simulink model "OFDM_Tx_Rx_InterpDec"  (R2020a)
settings: Solver=FixedStepDiscrete  StartTime=0.0  StopTime=inf  RelTol=1e-3
InitFcn:
  | % Set parameters
  | fs = 200e3;
  | 
  | % Load all required variables
  | load('read_addr_data');
  | load('read_addr_cp');
  | load('read_addr_pream');
  | load('read_addr_rx');
  | load('pilot');
  | load('LTSfreq');
  | load('STSfreq');
  | load('LTSread');
  | load('STSread');
  | load('bpsk');
  | load('qpsk');
  | load('qam16');
values from neighbouring files (symbols this model uses):
  bpsk = [0 0 1 1 1 1 0 0 1 0 1 0 ... (48 elements, 48x1)]    [bpsk.mat]
  qam16 = [12 5 10 3 14 8 1 10 8 7 2 13 ... (48 elements, 48x1)]    [qam16.mat]
  qpsk = [1 2 1 2 2 2 3 1 1 3 1 0 ... (48 elements, 48x1)]    [qpsk.mat]
  STSfreq = [0 0 0 0 0 0 0 0 1 0 0 0 ... (64 elements, 1x64)]    [STSfreq.mat]
undefined symbols (not defined in the file or in its folder): data3, designMultirateFIR, LTSfreq, LTSread, pilot, read_addr_cp, read_addr_data, read_addr_pream, read_addr_rx, STSread
libraries: hdlsllib x58, simulink x42, dspmlti4 x8, dsphdlxfrm x2, dsphdlmathfun x2, dsphdlsigops x1
(part 3 of 5)

== system OFDM_Tx_Rx_InterpDec/OFDMRx/Synchronisation/ControlSigGen/dataValidGen ==
  enb : Inport
  enb1 : Inport  Port=2
  AND : Logic  IconShape=distinctive  AllPortsSameDT=off  OutDataTypeStr=boolean
  Compare To Constant : simulink/Logic and Bit Operations/Compare To Constant  relop=>  const=15  OutDataTypeStr=boolean
  Delay : Delay  DelayLength=1
  HDL Counter : hdlsllib/Sources/HDL Counter  CountType=Count limited  CountInit=0  CountStep=1  CountMax=79  CountFromType=Initial value  CountFrom=0  CountResetPort=on  CountLoadPort=off  CountEnbPort=on  CountDirPort=off  CountDataType=Unsigned  CountWordLen=7  CountFracLen=0  CountSampTime=1
  NOT : Logic  Operator=NOT  IconShape=distinctive  AllPortsSameDT=off  OutDataTypeStr=boolean
  NOT1 : Logic  Operator=NOT  IconShape=distinctive  AllPortsSameDT=off  OutDataTypeStr=boolean
  y : Outport
  wires:
  HDL Counter/1 -> Compare To Constant/1
  NOT/1 -> HDL Counter/1
  Compare To Constant/1 -> y/1
  NOT1/1 -> AND/1
  AND/1 -> NOT/1, HDL Counter/2
  Delay/1 -> AND/2
  enb1/1 -> Delay/1
  enb/1 -> NOT1/1

== system OFDM_Tx_Rx_InterpDec/OFDMRx/Synchronisation/FineTimingSynch/Abs1 ==
  DataIn : Inport
  Add : Sum  OutDataTypeStr=fixdt(1,16,14)
  Complex to Real-Imag : ComplexToRealImag
  Delay{,1..3} (4 alike) : Delay  DelayLength=1
  Product : Product
  Product1 : Product
  Out1 : Outport  VectorParamsAs1DForOutWhenUnconnected=off
  wires:
  Add/1 -> Out1/1
  Complex to Real-Imag/1 -> Delay/1
  DataIn/1 -> Complex to Real-Imag/1
  Product/1 -> Delay2/1
  Product1/1 -> Delay3/1
  Complex to Real-Imag/2 -> Delay1/1
  Delay/1 -> Product/1, Product/2
  Delay1/1 -> Product1/2, Product1/1
  Delay2/1 -> Add/1
  Delay3/1 -> Add/2

== system OFDM_Tx_Rx_InterpDec/OFDMRx/Synchronisation/FineTimingSynch/Abs2 ==
  dataOut : Inport
  Add : Sum
  Complex to Real-Imag : ComplexToRealImag
  Delay{,1..3} (4 alike) : Delay  DelayLength=1
  Gain : Gain  Gain=1/64  OutDataTypeStr=double
  Product : Product
  Product1 : Product
  Out1 : Outport  VectorParamsAs1DForOutWhenUnconnected=off
  wires:
  Delay3/1 -> Add/2
  Delay2/1 -> Add/1
  Delay1/1 -> Product1/1, Product1/2
  Delay/1 -> Product/2, Product/1
  Complex to Real-Imag/2 -> Delay1/1
  Product1/1 -> Delay3/1
  Product/1 -> Delay2/1
  Add/1 -> Gain/1
  dataOut/1 -> Complex to Real-Imag/1
  Complex to Real-Imag/1 -> Delay/1
  Gain/1 -> Out1/1

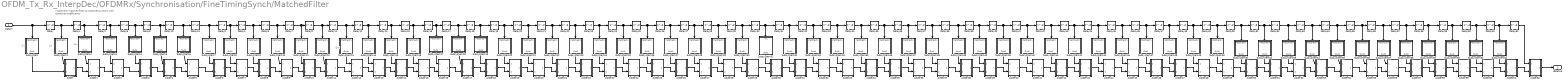
== system OFDM_Tx_Rx_InterpDec/OFDMRx/Synchronisation/FineTimingSynch/MatchedFilter ==
  note: -1+j
  note: 1+j
  note: 1-j
  note: -1-j
  note: Implement matched filter as pipleined systolic with
      | quantised coefficients
  dataIn : Inport
  Adder : Subsystem
  Adder1 : Subsystem
  Adder10 : Subsystem
  Adder11 : Subsystem
  Adder12 : Subsystem
  Adder13 : Subsystem
  Adder14 : Subsystem
  Adder15 : Subsystem
  Adder16 : Subsystem
  Adder17 : Subsystem
  Adder18 : Subsystem
  Adder19 : Subsystem
  Adder2 : Subsystem
  Adder20 : Subsystem
  Adder21 : Subsystem
  Adder22 : Subsystem
  Adder23 : Subsystem
  Adder24 : Subsystem
  Adder25 : Subsystem
  Adder26 : Subsystem
  Adder27 : Subsystem
  Adder28 : Subsystem
  Adder29 : Subsystem
  Adder3 : Subsystem
  Adder30 : Subsystem
  Adder31 : Subsystem
  Adder32 : Subsystem
  Adder33 : Subsystem
  Adder34 : Subsystem
  Adder35 : Subsystem
  Adder36 : Subsystem
  Adder37 : Subsystem
  Adder38 : Subsystem
  Adder39 : Subsystem
  Adder4 : Subsystem
  Adder40 : Subsystem
  Adder41 : Subsystem
  Adder42 : Subsystem
  Adder43 : Subsystem
  Adder44 : Subsystem
  Adder45 : Subsystem
  Adder46 : Subsystem
  Adder47 : Subsystem
  Adder48 : Subsystem
  Adder49 : Subsystem
  Adder5 : Subsystem
  Adder50 : Subsystem
  Adder51 : Subsystem
  Adder52 : Subsystem
  Adder53 : Subsystem
  Adder54 : Subsystem
  Adder55 : Subsystem
  Adder56 : Subsystem
  Adder57 : Subsystem
  Adder58 : Subsystem
  Adder59 : Subsystem
  Adder6 : Subsystem
  Adder60 : Subsystem
  Adder61 : Subsystem
  Adder62 : Subsystem
  Adder7 : Subsystem
  Adder8 : Subsystem
  Adder9 : Subsystem
  Delay{,1..62} (63 alike) : Delay
  Subsystem : Subsystem
  Subsystem1 : Subsystem
  Subsystem10 : Subsystem
  Subsystem11 : Subsystem
  Subsystem12 : Subsystem
  Subsystem13 : Subsystem
  Subsystem14 : Subsystem
  Subsystem15 : Subsystem
  Subsystem16 : Subsystem
  Subsystem17 : Subsystem
  Subsystem18 : Subsystem
  Subsystem19 : Subsystem
  Subsystem2 : Subsystem
  Subsystem20 : Subsystem
  Subsystem21 : Subsystem
  Subsystem22 : Subsystem
  Subsystem23 : Subsystem
  Subsystem24 : Subsystem
  Subsystem25 : Subsystem
  Subsystem26 : Subsystem
  Subsystem27 : Subsystem
  Subsystem28 : Subsystem
  Subsystem29 : Subsystem
  Subsystem3 : Subsystem
  Subsystem30 : Subsystem
  Subsystem31 : Subsystem
  Subsystem32 : Subsystem
  Subsystem33 : Subsystem
  Subsystem34 : Subsystem
  Subsystem35 : Subsystem
  Subsystem36 : Subsystem
  Subsystem37 : Subsystem
  Subsystem38 : Subsystem
  Subsystem39 : Subsystem
  Subsystem4 : Subsystem
  Subsystem40 : Subsystem
  Subsystem41 : Subsystem
  Subsystem42 : Subsystem
  Subsystem43 : Subsystem
  Subsystem44 : Subsystem
  Subsystem45 : Subsystem
  Subsystem46 : Subsystem
  Subsystem47 : Subsystem
  Subsystem48 : Subsystem
  Subsystem5 : Subsystem
  Subsystem50 : Subsystem
  Subsystem51 : Subsystem
  Subsystem52 : Subsystem
  Subsystem53 : Subsystem
  Subsystem54 : Subsystem
  Subsystem55 : Subsystem
  Subsystem56 : Subsystem
  Subsystem57 : Subsystem
  Subsystem58 : Subsystem
  Subsystem59 : Subsystem
  Subsystem6 : Subsystem
  Subsystem60 : Subsystem
  Subsystem61 : Subsystem
  Subsystem62 : Subsystem
  Subsystem63 : Subsystem
  Subsystem7 : Subsystem
  Subsystem8 : Subsystem
  Subsystem9 : Subsystem
  dataOut : Outport  VectorParamsAs1DForOutWhenUnconnected=off
  wires:
  Adder62/1(Out1) -> dataOut/1
  Adder61/1(Out1) -> Adder62/2(In2)
  Delay61/1 -> Subsystem62/1(MatchedIn), Delay62/1
  Adder60/1(Out1) -> Adder61/2(In2)
  Delay60/1 -> Subsystem61/1(MatchedIn), Delay61/1
  Adder59/1(Out1) -> Adder60/2(In2)
  Delay59/1 -> Delay60/1, Subsystem60/1(MatchedIn)
  Adder58/1(Out1) -> Adder59/2(In2)
  Delay58/1 -> Subsystem59/1(MatchedIn), Delay59/1
  Adder57/1(Out1) -> Adder58/2(In2)
  Delay57/1 -> Delay58/1, Subsystem58/1(MatchedIn)
  Adder56/1(Out1) -> Adder57/2(In2)
  Delay56/1 -> Subsystem57/1(MatchedIn), Delay57/1
  Adder55/1(Out1) -> Adder56/2(In2)
  Delay55/1 -> Subsystem56/1(MatchedIn), Delay56/1
  Adder54/1(Out1) -> Adder55/2(In2)
  Delay54/1 -> Subsystem55/1(MatchedIn), Delay55/1
  Adder53/1(Out1) -> Adder54/2(In2)
  Delay53/1 -> Subsystem54/1(MatchedIn), Delay54/1
  Adder52/1(Out1) -> Adder53/2(In2)
  Delay52/1 -> Subsystem53/1(MatchedIn), Delay53/1
  Adder51/1(Out1) -> Adder52/2(In2)
  Delay51/1 -> Delay52/1, Subsystem52/1(MatchedIn)
  Adder50/1(Out1) -> Adder51/2(In2)
  Delay50/1 -> Delay51/1, Subsystem51/1(MatchedIn)
  Adder49/1(Out1) -> Adder50/2(In2)
  Delay49/1 -> Delay50/1, Subsystem50/1(MatchedIn)
  Adder48/1(Out1) -> Adder49/2(In2)
  Delay48/1 -> Subsystem45/1(MatchedIn), Delay49/1
  Adder47/1(Out1) -> Adder48/2(In2)
  Delay47/1 -> Subsystem48/1(MatchedIn), Delay48/1
  Adder46/1(Out1) -> Adder47/2(In2)
  Delay46/1 -> Subsystem47/1(MatchedIn), Delay47/1
  Adder45/1(Out1) -> Adder46/2(In2)
  Delay45/1 -> Subsystem46/1(MatchedIn), Delay46/1
  Adder44/1(Out1) -> Adder45/2(In2)
  Delay44/1 -> Subsystem44/1(MatchedIn), Delay45/1
  Adder43/1(Out1) -> Adder44/2(In2)
  Delay43/1 -> Subsystem41/1(MatchedIn), Delay44/1
  Adder42/1(Out1) -> Adder43/2(In2)
  Delay42/1 -> Subsystem43/1(MatchedIn), Delay43/1
  Adder41/1(Out1) -> Adder42/2(In2)
  Delay41/1 -> Subsystem42/1(MatchedIn), Delay42/1
  Adder40/1(Out1) -> Adder41/2(In2)
  Delay40/1 -> Subsystem35/1(MatchedIn), Delay41/1
  Adder39/1(Out1) -> Adder40/2(In2)
  Delay39/1 -> Delay40/1, Subsystem40/1(MatchedIn)
  Adder38/1(Out1) -> Adder39/2(In2)
  Delay38/1 -> Subsystem39/1(MatchedIn), Delay39/1
  Adder37/1(Out1) -> Adder38/2(In2)
  Delay37/1 -> Delay38/1, Subsystem38/1(MatchedIn)
  Adder36/1(Out1) -> Adder37/2(In2)
  Delay36/1 -> Subsystem37/1(MatchedIn), Delay37/1
  Adder35/1(Out1) -> Adder36/2(In2)
  Delay35/1 -> Subsystem36/1(MatchedIn), Delay36/1
  Adder34/1(Out1) -> Adder35/2(In2)
  Delay34/1 -> Subsystem63/1(MatchedIn), Delay35/1
  Adder33/1(Out1) -> Adder34/2(In2)
  Delay33/1 -> Subsystem34/1(MatchedIn), Delay34/1
  Adder32/1(Out1) -> Adder33/2(In2)
  Delay32/1 -> Delay33/1, Subsystem33/1(MatchedIn)
  Adder31/1(Out1) -> Adder32/2(In2)
  Delay31/1 -> Subsystem32/1(MatchedIn), Delay32/1
  Adder30/1(Out1) -> Adder31/2(In2)
  Delay30/1 -> Subsystem31/1(In1), Delay31/1
  Adder29/1(Out1) -> Adder30/2(In2)
  Delay29/1 -> Delay30/1, Subsystem30/1(MatchedIn)
  Adder28/1(Out1) -> Adder29/2(In2)
  Delay28/1 -> Subsystem29/1(MatchedIn), Delay29/1
  Adder27/1(Out1) -> Adder28/2(In2)
  Delay27/1 -> Subsystem28/1(MatchedIn), Delay28/1
  Adder26/1(Out1) -> Adder27/2(In2)
  Delay26/1 -> Subsystem27/1(MatchedIn), Delay27/1
  Adder25/1(Out1) -> Adder26/2(In2)
  Delay25/1 -> Delay26/1, Subsystem26/1(MatchedIn)
  Adder24/1(Out1) -> Adder25/2(In2)
  Delay24/1 -> Subsystem25/1(MatchedIn), Delay25/1
  Adder23/1(Out1) -> Adder24/2(In2)
  Adder22/1(Out1) -> Adder23/2(In2)
  Delay21/1 -> Subsystem22/1(MatchedIn), Delay22/1
  Delay22/1 -> Subsystem23/1(MatchedIn), Delay23/1
  Adder21/1(Out1) -> Adder22/2(In2)
  Adder20/1(Out1) -> Adder21/2(In2)
  Delay20/1 -> Subsystem21/1(MatchedIn), Delay21/1
  Adder19/1(Out1) -> Adder20/2(In2)
  Delay19/1 -> Subsystem20/1(MatchedIn), Delay20/1
  Adder18/1(Out1) -> Adder19/2(In2)
  Adder17/1(Out1) -> Adder18/2(In2)
  Delay18/1 -> Subsystem19/1(MatchedIn), Delay19/1
  Delay17/1 -> Subsystem18/1(MatchedIn), Delay18/1
  Adder16/1(Out1) -> Adder17/2(In2)
  Adder15/1(Out1) -> Adder16/2(In2)
  Delay16/1 -> Subsystem17/1(MatchedIn), Delay17/1
  Delay15/1 -> Subsystem16/1(MatchedIn), Delay16/1
  Adder14/1(Out1) -> Adder15/2(In2)
  Adder13/1(Out1) -> Adder14/2(In2)
  Delay14/1 -> Subsystem15/1(MatchedIn), Delay15/1
  Adder12/1(Out1) -> Adder13/2(In2)
  Delay12/1 -> Subsystem14/1(MatchedIn), Delay14/1
  Adder11/1(Out1) -> Adder12/2(In2)
  Delay11/1 -> Subsystem13/1(MatchedIn), Delay12/1
  Adder10/1(Out1) -> Adder11/2(In2)
  Delay9/1 -> Subsystem12/1(MatchedIn), Delay11/1
  Adder9/1(Out1) -> Adder10/2(In2)
  Delay7/1 -> Subsystem11/1(MatchedIn), Delay9/1
  Delay5/1 -> Subsystem10/1(MatchedIn), Delay7/1
  Adder8/1(Out1) -> Adder9/2(In2)
  Adder7/1(Out1) -> Adder8/2(In2)
  Delay4/1 -> Subsystem9/1(MatchedIn), Delay5/1
  Adder6/1(Out1) -> Adder7/2(In2)
  Delay3/1 -> Subsystem8/1(MatchedIn), Delay4/1
  Adder5/1(Out1) -> Adder6/2(In2)
  Adder4/1(Out1) -> Adder5/2(In2)
  Adder3/1(Out1) -> Adder4/2(In2)
  Adder2/1(Out1) -> Adder3/2(In2)
  Adder1/1(Out1) -> Adder2/2(In2)
  Adder/1(Out1) -> Adder1/2(In2)
  Delay13/1 -> Subsystem7/1(MatchedIn), Delay3/1
  Delay10/1 -> Subsystem6/1(MatchedIn), Delay13/1
  Delay8/1 -> Subsystem5/1(MatchedIn), Delay10/1
  Delay6/1 -> Subsystem4/1(MatchedIn), Delay8/1
  Delay2/1 -> Subsystem3/1(MatchedIn), Delay6/1
  Delay1/1 -> Subsystem2/1(MatchedIn), Delay2/1
  Delay/1 -> Subsystem1/1(MatchedIn), Delay1/1
  dataIn/1 -> Delay/1, Subsystem/1(MatchedIn)
  Subsystem/1(Out1) -> Adder/2(In2)
  Subsystem1/1(Out1) -> Adder/1(In1)
  Subsystem3/1(Out1) -> Adder2/1(In1)
  Subsystem4/1(Out1) -> Adder3/1(In1)
  Subsystem5/1(Out1) -> Adder4/1(In1)
  Subsystem6/1(Out1) -> Adder5/1(In1)
  Subsystem7/1(Out1) -> Adder6/1(In1)
  Subsystem8/1(Out1) -> Adder7/1(In1)
  Subsystem9/1(Out1) -> Adder8/1(In1)
  Subsystem10/1(Out1) -> Adder9/1(In1)
  Subsystem11/1(Out1) -> Adder10/1(In1)
  Subsystem12/1(Out1) -> Adder11/1(In1)
  Subsystem13/1(Out1) -> Adder12/1(In1)
  Subsystem14/1(Out1) -> Adder13/1(In1)
  Subsystem15/1(Out1) -> Adder14/1(In1)
  Subsystem16/1(Out1) -> Adder15/1(In1)
  Subsystem17/1(Out1) -> Adder16/1(In1)
  Subsystem18/1(Out1) -> Adder17/1(In1)
  Subsystem19/1(Out1) -> Adder18/1(In1)
  Subsystem20/1(Out1) -> Adder19/1(In1)
  Subsystem21/1(Out1) -> Adder20/1(In1)
  Subsystem22/1(Out1) -> Adder21/1(In1)
  Subsystem23/1(Out1) -> Adder22/1(In1)
  Delay23/1 -> Subsystem24/1(MatchedIn), Delay24/1
  Subsystem24/1(Out1) -> Adder23/1(In1)
  Subsystem25/1(Out1) -> Adder24/1(In1)
  Subsystem26/1(Out1) -> Adder25/1(In1)
  Subsystem27/1(Out1) -> Adder26/1(In1)
  Subsystem28/1(Out1) -> Adder27/1(In1)
  Subsystem29/1(Out1) -> Adder28/1(In1)
  Subsystem30/1(Out1) -> Adder29/1(In1)
  Subsystem31/1(Out1) -> Adder30/1(In1)
  Subsystem32/1(Out1) -> Adder31/1(In1)
  Subsystem33/1(Out1) -> Adder32/1(In1)
  Subsystem34/1(Out1) -> Adder33/1(In1)
  Subsystem63/1(Out1) -> Adder34/1(In1)
  Subsystem36/1(Out1) -> Adder35/1(In1)
  Subsystem37/1(Out1) -> Adder36/1(In1)
  Subsystem38/1(Out1) -> Adder37/1(In1)
  Subsystem39/1(Out1) -> Adder38/1(In1)
  Subsystem40/1(Out1) -> Adder39/1(In1)
  Subsystem35/1(Out1) -> Adder40/1(In1)
  Subsystem42/1(Out1) -> Adder41/1(In1)
  Subsystem43/1(Out1) -> Adder42/1(In1)
  Subsystem41/1(Out1) -> Adder43/1(In1)
  Subsystem44/1(Out1) -> Adder44/1(In1)
  Subsystem46/1(Out1) -> Adder45/1(In1)
  Subsystem47/1(Out1) -> Adder46/1(In1)
  Subsystem48/1(Out1) -> Adder47/1(In1)
  Subsystem45/1(Out1) -> Adder48/1(In1)
  Subsystem50/1(Out1) -> Adder49/1(In1)
  Subsystem51/1(Out1) -> Adder50/1(In1)
  Subsystem52/1(Out1) -> Adder51/1(In1)
  Subsystem53/1(Out1) -> Adder52/1(In1)
  Subsystem54/1(Out1) -> Adder53/1(In1)
  Subsystem55/1(Out1) -> Adder54/1(In1)
  Subsystem56/1(Out1) -> Adder55/1(In1)
  Subsystem57/1(Out1) -> Adder56/1(In1)
  Subsystem58/1(Out1) -> Adder57/1(In1)
  Subsystem59/1(Out1) -> Adder58/1(In1)
  Subsystem60/1(Out1) -> Adder59/1(In1)
  Subsystem61/1(Out1) -> Adder60/1(In1)
  Subsystem62/1(Out1) -> Adder61/1(In1)
  Delay62/1 -> Adder62/1(In1)
  Subsystem2/1(Out1) -> Adder1/1(In1)

== system OFDM_Tx_Rx_InterpDec/OFDMRx/Synchronisation/FineTimingSynch/MovingAvg ==
  DataIn : Inport
  Add : Sum  Inputs=-+  AccumDataTypeStr=fixdt(1,24,14)
  Add1 : Sum  AccumDataTypeStr=fixdt(1,24,14)
  Delay1 : Delay  DelayLength=64
  Delay2 : Delay  DelayLength=1
  Delay3 : Delay  DelayLength=1
  Delay4 : Delay  DelayLength=1
  Out1 : Outport  VectorParamsAs1DForOutWhenUnconnected=off
  wires:
  Delay3/1 -> Add/2, Delay1/1
  Add/1 -> Add1/2
  Delay1/1 -> Add/1
  DataIn/1 -> Delay3/1
  Add1/1 -> Delay2/1
  Delay2/1 -> Delay4/1, Add1/1
  Delay4/1 -> Out1/1

== system OFDM_Tx_Rx_InterpDec/OFDMRx/Synchronisation/FineTimingSynch/threshCompare ==
  In1 : Inport
  In2 : Inport  Port=2
  Constant1 : Constant  OutDataTypeStr=boolean  SampleTime=1/fs
  Constant2 : Constant  Value=0  OutDataTypeStr=boolean  SampleTime=1/fs
  Relational Operator : RelationalOperator  Operator=>  OutDataTypeStr=boolean  RndMeth=Simplest
  Unit Delay Enabled Resettable Synchronous : hdlsllib/Discrete/Unit Delay Enabled Resettable Synchronous  InitialCondition=0.0  SampleTime=-1
      settings: SourceProductBaseCode=SL
  Out1 : Outport
  wires:
  Constant1/1 -> Unit Delay Enabled Resettable Synchronous/1
  In1/1 -> Relational Operator/1
  Relational Operator/1 -> Unit Delay Enabled Resettable Synchronous/2
  Unit Delay Enabled Resettable Synchronous/1 -> Out1/1
  Constant2/1 -> Unit Delay Enabled Resettable Synchronous/3
  In2/1 -> Relational Operator/2

== system OFDM_Tx_Rx_InterpDec/OFDMRx/Synchronisation/FrameDetect/RsingEdge ==
  In1 : Inport
  Constant : Constant  OutDataTypeStr=boolean  SampleTime=1/fs
  Constant1 : Constant  Value=0  OutDataTypeStr=boolean  SampleTime=1/fs
  Delay : Delay  DelayLength=1
  Relational Operator : RelationalOperator  Operator=>  OutDataTypeStr=boolean  RndMeth=Nearest
  Unit Delay Enabled Resettable Synchronous : hdlsllib/Discrete/Unit Delay Enabled Resettable Synchronous  InitialCondition=0.0  SampleTime=-1
      settings: SourceProductBaseCode=SL
  Out1 : Outport  VectorParamsAs1DForOutWhenUnconnected=off
  wires:
  Relational Operator/1 -> Unit Delay Enabled Resettable Synchronous/2
  Delay/1 -> Relational Operator/2
  In1/1 -> Delay/1, Relational Operator/1
  Unit Delay Enabled Resettable Synchronous/1 -> Out1/1
  Constant/1 -> Unit Delay Enabled Resettable Synchronous/1
  Constant1/1 -> Unit Delay Enabled Resettable Synchronous/3

== system OFDM_Tx_Rx_InterpDec/OFDMRx/Synchronisation/SchmidlCoxMetric /Abs2 ==
  Abs2In : Inport
  Add : Sum  OutDataTypeStr=fixdt(0,25,23)
  Complex to Real-Imag : ComplexToRealImag
  Delay{1..4} (4 alike) : Delay  DelayLength=1
  Delay5 : Delay
  Product : Product  OutDataTypeStr=fixdt(0,25,23)
  Product1 : Product  OutDataTypeStr=fixdt(0,25,23)
  Abs2Out : Outport  VectorParamsAs1DForOutWhenUnconnected=off
  wires:
  Delay5/1 -> Abs2Out/1
  Delay4/1 -> Add/2
  Delay3/1 -> Add/1
  Delay2/1 -> Product1/1, Product1/2
  Delay1/1 -> Product/2, Product/1
  Add/1 -> Delay5/1
  Product1/1 -> Delay4/1
  Product/1 -> Delay3/1
  Complex to Real-Imag/2 -> Delay2/1
  Complex to Real-Imag/1 -> Delay1/1
  Abs2In/1 -> Complex to Real-Imag/1

== system OFDM_Tx_Rx_InterpDec/OFDMRx/Synchronisation/SchmidlCoxMetric /AutoCorr ==
  AcorrIn : Inport
  Delay : Delay  DelayLength=16
  Delay{1..5} (5 alike) : Delay  DelayLength=1
  Math Function : Math  Operator=conj  SignedPower=on  RndMeth=Zero  SaturateOnIntegerOverflow=on
  Product : Product  OutDataTypeStr=fixdt(1,25,23)
  AcorrOut : Outport  VectorParamsAs1DForOutWhenUnconnected=off
  wires:
  Delay5/1 -> Delay2/1
  Delay4/1 -> Product/2
  Delay3/1 -> Product/1
  Delay2/1 -> AcorrOut/1
  Delay1/1 -> Delay3/1, Delay/1
  Delay/1 -> Math Function/1
  Product/1 -> Delay5/1
  Math Function/1 -> Delay4/1
  AcorrIn/1 -> Delay1/1

== system OFDM_Tx_Rx_InterpDec/OFDMRx/Synchronisation/SchmidlCoxMetric /CIC_ma ==
  note: The averaging window is set to 64 samples i.e.
      | 4x repetitions of the L-STF. Using a larger averaging
      | window improves the coarse CFO estimate. This
      | approach leaves 6x L-STF repetitions for AGC convergence.
  In1 : Inport
  Add : Sum  Inputs=-+  AccumDataTypeStr=fixdt(1,33,23)
  Add1 : Sum  AccumDataTypeStr=fixdt(1,33,23)
  Data Type Conversion : DataTypeConversion  OutDataTypeStr=fixdt(1,18,16)
  Delay1 : Delay  DelayLength=48
  Delay2 : Delay  DelayLength=1
  Delay3 : Delay  DelayLength=1
  Delay4 : Delay  DelayLength=1
  Out1 : Outport  VectorParamsAs1DForOutWhenUnconnected=off
  wires:
  Data Type Conversion/1 -> Out1/1
  Delay4/1 -> Data Type Conversion/1
  Delay3/1 -> Delay1/1, Add/2
  Delay2/1 -> Add1/1, Delay4/1
  Add1/1 -> Delay2/1
  In1/1 -> Delay3/1
  Delay1/1 -> Add/1
  Add/1 -> Add1/2

== system OFDM_Tx_Rx_InterpDec/OFDMRx/Synchronisation/SchmidlCoxMetric /CIC_ma1 ==
  In1 : Inport
  Add : Sum  Inputs=-+  AccumDataTypeStr=fixdt(1,33,23)
  Add1 : Sum  AccumDataTypeStr=fixdt(1,33,23)
  Data Type Conversion : DataTypeConversion  OutDataTypeStr=fixdt(1,18,15)
  Delay1 : Delay  DelayLength=48
  Delay2 : Delay  DelayLength=1
  Delay3 : Delay  DelayLength=1
  Delay4 : Delay  DelayLength=1
  Out1 : Outport  VectorParamsAs1DForOutWhenUnconnected=off
  wires:
  Data Type Conversion/1 -> Out1/1
  Delay4/1 -> Data Type Conversion/1
  Delay3/1 -> Add/2, Delay1/1
  Add/1 -> Add1/2
  Delay1/1 -> Add/1
  In1/1 -> Delay3/1
  Add1/1 -> Delay2/1
  Delay2/1 -> Delay4/1, Add1/1

== system OFDM_Tx_Rx_InterpDec/OFDMRx/Synchronisation/SchmidlCoxMetric /MagPhase ==
  dataIn : Inport
  Complex to Magnitude-Angle HDL Optimized : dsphdlmathfun/Complex to Magnitude-Angle HDL Optimized  NumIterationsSource=Property  NumIterations=10  OutputFormat=Magnitude and angle  AngleFormat=Normalized  ScaleOutput=on  SimulateUsing=Code generation
      settings: SourceProductBaseCode=DS
  Constant : Constant  OutDataTypeStr=boolean  SampleTime=1/fs
  Data Type Conversion : DataTypeConversion  OutDataTypeStr=fixdt(1,18,16)
  Data Type Conversion1 : DataTypeConversion  OutDataTypeStr=fixdt(1,25,22)
  Terminator1 : Terminator
  Phase : Outport  VectorParamsAs1DForOutWhenUnconnected=off
  Mag : Outport  Port=2  VectorParamsAs1DForOutWhenUnconnected=off
  wires:
  Data Type Conversion1/1 -> Phase/1
  Data Type Conversion/1 -> Mag/1
  Complex to Magnitude-Angle HDL Optimized/2 -> Data Type Conversion1/1
  Complex to Magnitude-Angle HDL Optimized/3 -> Terminator1/1
  Complex to Magnitude-Angle HDL Optimized/1 -> Data Type Conversion/1
  dataIn/1 -> Complex to Magnitude-Angle HDL Optimized/1
  Constant/1 -> Complex to Magnitude-Angle HDL Optimized/2

== system OFDM_Tx_Rx_InterpDec/OFDMRx/Synchronisation/SchmidlCoxMetric /Sq ==
  In1 : Inport
  Delay : Delay  DelayLength=1
  Delay1 : Delay  DelayLength=1
  Product : Product
  Out1 : Outport  VectorParamsAs1DForOutWhenUnconnected=off
  wires:
  Delay1/1 -> Out1/1
  Delay/1 -> Product/2, Product/1
  Product/1 -> Delay1/1
  In1/1 -> Delay/1

== system OFDM_Tx_Rx_InterpDec/OFDMRx/Synchronisation/SchmidlCoxMetric /Sq1 ==
  In1 : Inport
  Delay : Delay  DelayLength=1
  Delay1 : Delay  DelayLength=1
  Product : Product
  Out1 : Outport  VectorParamsAs1DForOutWhenUnconnected=off
  wires:
  In1/1 -> Delay/1
  Product/1 -> Delay1/1
  Delay/1 -> Product/1, Product/2
  Delay1/1 -> Out1/1

== system OFDM_Tx_Rx_InterpDec/OFDMRx/Synchronisation/SchmidlCoxMetric /ThreshMult ==
  In1 : Inport
  ThreshMult : Gain  Gain=0.5  OutDataTypeStr=fixdt(1,33,23)
  Out1 : Outport  VectorParamsAs1DForOutWhenUnconnected=off
  wires:
  In1/1 -> ThreshMult/1
  ThreshMult/1 -> Out1/1

== system OFDM_Tx_Rx_InterpDec/OFDMTx/CPAdd/DataExtend/READ_CTRL2 ==
  In1 : Inport
  In2 : Inport  Port=2
  Constant : Constant  Value=0  OutDataTypeStr=fixdt(0,8,0)  SampleTime=1/fs
  Switch : Switch  Criteria=u2 ~= 0
  Out1 : Outport  VectorParamsAs1DForOutWhenUnconnected=off
  wires:
  Constant/1 -> Switch/3
  In2/1 -> Switch/2
  In1/1 -> Switch/1
  Switch/1 -> Out1/1

== system OFDM_Tx_Rx_InterpDec/OFDMTx/CPAdd/LTFExtend/LTFValidGen ==
  In1 : Inport
  AND : Logic  IconShape=distinctive  AllPortsSameDT=off  OutDataTypeStr=boolean
  AND1 : Logic  IconShape=distinctive  AllPortsSameDT=off  OutDataTypeStr=boolean
  Compare To Constant : simulink/Logic and Bit Operations/Compare To Constant  relop=>=  const=160  OutDataTypeStr=boolean
  Compare To Constant1 : simulink/Logic and Bit Operations/Compare To Constant  relop=<=  const=319  OutDataTypeStr=boolean
  HDL Counter : hdlsllib/Sources/HDL Counter  CountType=Count limited  CountInit=0  CountStep=1  CountMax=319  CountFromType=Initial value  CountFrom=0  CountResetPort=on  CountLoadPort=off  CountEnbPort=on  CountDirPort=off  CountDataType=Unsigned  CountWordLen=9  CountFracLen=0  CountSampTime=1
  NOT : Logic  Operator=NOT  IconShape=distinctive  AllPortsSameDT=off  OutDataTypeStr=boolean
  Out1 : Outport  VectorParamsAs1DForOutWhenUnconnected=off
  wires:
  Compare To Constant/1 -> AND/1
  In1/1 -> NOT/1, AND1/2, HDL Counter/2
  HDL Counter/1 -> Compare To Constant1/1, Compare To Constant/1
  Compare To Constant1/1 -> AND/2
  AND1/1 -> Out1/1
  AND/1 -> AND1/1
  NOT/1 -> HDL Counter/1

== system OFDM_Tx_Rx_InterpDec/OFDMTx/CPAdd/LTFExtend/READ_CTRL ==
  In1 : Inport
  In2 : Inport  Port=2
  Constant : Constant  Value=0  OutDataTypeStr=fixdt(0,8,0)  SampleTime=1/fs
  Switch : Switch  Criteria=u2 ~= 0
  Out1 : Outport  VectorParamsAs1DForOutWhenUnconnected=off
  wires:
  Switch/1 -> Out1/1
  In1/1 -> Switch/1
  In2/1 -> Switch/2
  Constant/1 -> Switch/3

== system OFDM_Tx_Rx_InterpDec/OFDMTx/CPAdd/STFExtend/READ_CTRL ==
  In1 : Inport
  In2 : Inport  Port=2
  Constant : Constant  Value=0  OutDataTypeStr=fixdt(0,8,0)  SampleTime=1/fs
  Switch : Switch  Criteria=u2 ~= 0
  Out1 : Outport  VectorParamsAs1DForOutWhenUnconnected=off
  wires:
  Constant/1 -> Switch/3
  In2/1 -> Switch/2
  In1/1 -> Switch/1
  Switch/1 -> Out1/1

== system OFDM_Tx_Rx_InterpDec/OFDMTx/CPAdd/STFExtend/STFValidGen ==
  In1 : Inport
  AND : Logic  IconShape=distinctive  AllPortsSameDT=off  OutDataTypeStr=boolean
  AND1 : Logic  IconShape=distinctive  AllPortsSameDT=off  OutDataTypeStr=boolean
  Compare To Constant : simulink/Logic and Bit Operations/Compare To Constant  relop=>=  const=0  OutDataTypeStr=boolean
  Compare To Constant1 : simulink/Logic and Bit Operations/Compare To Constant  relop=<=  const=159  OutDataTypeStr=boolean
  HDL Counter : hdlsllib/Sources/HDL Counter  CountType=Count limited  CountInit=0  CountStep=1  CountMax=319  CountFromType=Initial value  CountFrom=0  CountResetPort=on  CountLoadPort=off  CountEnbPort=on  CountDirPort=off  CountDataType=Unsigned  CountWordLen=9  CountFracLen=0  CountSampTime=1
  NOT : Logic  Operator=NOT  IconShape=distinctive  AllPortsSameDT=off  OutDataTypeStr=boolean
  Out1 : Outport  VectorParamsAs1DForOutWhenUnconnected=off
  wires:
  Compare To Constant/1 -> AND/1
  In1/1 -> NOT/1, AND1/2, HDL Counter/2
  HDL Counter/1 -> Compare To Constant1/1, Compare To Constant/1
  Compare To Constant1/1 -> AND/2
  AND1/1 -> Out1/1
  AND/1 -> AND1/1
  NOT/1 -> HDL Counter/1

== system OFDM_Tx_Rx_InterpDec/OFDMTx/ControlSignalGenerator/PreamValidGen/RisingEdge ==
  In1 : Inport
  Delay : Delay  DelayLength=1
  Relational Operator : RelationalOperator  Operator=>  OutDataTypeStr=boolean  RndMeth=Nearest
  Out1 : Outport
  wires:
  Relational Operator/1 -> Out1/1
  Delay/1 -> Relational Operator/2
  In1/1 -> Delay/1, Relational Operator/1

== system OFDM_Tx_Rx_InterpDec/OFDMTx/DataGenerator/PilotGen/ToComplex1 ==
  In1 : Inport
  Constant1 : Constant  Value=0  OutDataTypeStr=fixdt(1,16,14)  SampleTime=1/fs
  Real-Imag to Complex : RealImagToComplex
  PilotOut : Outport  VectorParamsAs1DForOutWhenUnconnected=off
  wires:
  Constant1/1 -> Real-Imag to Complex/2
  In1/1 -> Real-Imag to Complex/1
  Real-Imag to Complex/1 -> PilotOut/1

== system OFDM_Tx_Rx_InterpDec/OFDMTx/DataGenerator/SymbolsGen/BPSKmap ==
  bits : Inport
  validIn : Inport  Port=2
  Constant : Constant  Value=complex(-1+0*1i)  VectorParams1D=off  OutDataTypeStr=fixdt(1,16,14)  SampleTime=1/fs
  Constant1 : Constant  Value=complex(1+0*1i)  VectorParams1D=off  OutDataTypeStr=fixdt(1,16,14)  SampleTime=1/fs
  Constant4 : Constant  Value=complex(0)  VectorParams1D=off  OutDataTypeStr=fixdt(1,16,14)  SampleTime=1/fs
  Multiport Switch : MultiPortSwitch  DataPortOrder=Zero-based contiguous  Inputs=2  zeroidx=on
  Switch : Switch  Criteria=u2 ~= 0
  BPSKOut : Outport  VectorParamsAs1DForOutWhenUnconnected=off
  wires:
  Switch/1 -> BPSKOut/1
  Constant4/1 -> Switch/3
  Multiport Switch/1 -> Switch/1
  validIn/1 -> Switch/2
  Constant1/1 -> Multiport Switch/3
  Constant/1 -> Multiport Switch/2
  bits/1 -> Multiport Switch/1

== system OFDM_Tx_Rx_InterpDec/OFDMTx/DataGenerator/SymbolsGen/DataGenerator ==
  ready : Inport
  1-D Lookup Table : Lookup_n-D  NumberOfTableDimensions=1  LookupTableObject=''  BreakpointsForDimension1=0:47  BreakpointsForDimension1FirstPoint=10  BreakpointsForDimension2FirstPoint=10  BreakpointsForDimension1Spacing=12  BreakpointsForDimension2Spacing=12  IndexSearchMethod=Evenly spaced points  Table=bpsk  TableDataTypeStr=fixdt(0,1,0)  InterpMethod=Flat  DiagnosticForOutOfRangeInput=Error  InternalRulePriority=Speed  OutDataTypeStr=fixdt(0,1,0)  RndMeth=Simplest  InputSameDT=on
  HDL Counter : hdlsllib/Sources/HDL Counter  CountType=Count limited  CountInit=0  CountStep=1  CountMax=47  CountFromType=Initial value  CountFrom=0  CountResetPort=off  CountLoadPort=off  CountEnbPort=on  CountDirPort=off  CountDataType=Unsigned  CountWordLen=6  CountFracLen=0  CountSampTime=1
  bits : Outport  VectorParamsAs1DForOutWhenUnconnected=off
  validOut : Outport  Port=2  VectorParamsAs1DForOutWhenUnconnected=off
  wires:
  HDL Counter/1 -> 1-D Lookup Table/1
  ready/1 -> validOut/1, HDL Counter/1
  1-D Lookup Table/1 -> bits/1

== system OFDM_Tx_Rx_InterpDec/OFDMTx/DataGenerator/SymbolsGen/DataGenerator1 ==
  ready : Inport
  1-D Lookup Table : Lookup_n-D  NumberOfTableDimensions=1  LookupTableObject=''  BreakpointsForDimension1=0:47  BreakpointsForDimension1FirstPoint=10  BreakpointsForDimension2FirstPoint=10  BreakpointsForDimension1Spacing=12  BreakpointsForDimension2Spacing=12  IndexSearchMethod=Evenly spaced points  Table=qpsk  TableDataTypeStr=fixdt(0,2,0)  InterpMethod=Flat  DiagnosticForOutOfRangeInput=Error  InternalRulePriority=Speed  OutDataTypeStr=fixdt(0,2,0)  RndMeth=Simplest  InputSameDT=on
  HDL Counter : hdlsllib/Sources/HDL Counter  CountType=Count limited  CountInit=0  CountStep=1  CountMax=47  CountFromType=Initial value  CountFrom=0  CountResetPort=off  CountLoadPort=off  CountEnbPort=on  CountDirPort=off  CountDataType=Unsigned  CountWordLen=6  CountFracLen=0  CountSampTime=1
  bits : Outport  VectorParamsAs1DForOutWhenUnconnected=off
  validOut : Outport  Port=2  VectorParamsAs1DForOutWhenUnconnected=off
  wires:
  1-D Lookup Table/1 -> bits/1
  ready/1 -> HDL Counter/1, validOut/1
  HDL Counter/1 -> 1-D Lookup Table/1

== system OFDM_Tx_Rx_InterpDec/OFDMTx/DataGenerator/SymbolsGen/DataGenerator2 ==
  ready : Inport
  1-D Lookup Table : Lookup_n-D  NumberOfTableDimensions=1  LookupTableObject=''  BreakpointsForDimension1=0:23  BreakpointsForDimension1FirstPoint=10  BreakpointsForDimension2FirstPoint=10  BreakpointsForDimension1Spacing=12  BreakpointsForDimension2Spacing=12  IndexSearchMethod=Evenly spaced points  Table=data3  TableDataTypeStr=fixdt(0,4,0)  InterpMethod=Flat  DiagnosticForOutOfRangeInput=Error  InternalRulePriority=Speed  OutDataTypeStr=fixdt(0,4,0)  RndMeth=Simplest  InputSameDT=on
  HDL Counter : hdlsllib/Sources/HDL Counter  CountType=Count limited  CountInit=0  CountStep=1  CountMax=23  CountFromType=Initial value  CountFrom=0  CountResetPort=off  CountLoadPort=off  CountEnbPort=on  CountDirPort=off  CountDataType=Unsigned  CountWordLen=5  CountFracLen=0  CountSampTime=1
  ints : Outport  VectorParamsAs1DForOutWhenUnconnected=off
  validOut : Outport  Port=2  VectorParamsAs1DForOutWhenUnconnected=off
  wires:
  1-D Lookup Table/1 -> ints/1
  ready/1 -> validOut/1, HDL Counter/1
  HDL Counter/1 -> 1-D Lookup Table/1

== system OFDM_Tx_Rx_InterpDec/OFDMTx/DataGenerator/SymbolsGen/DataGenerator3 ==
  ready : Inport
  1-D Lookup Table : Lookup_n-D  NumberOfTableDimensions=1  LookupTableObject=''  BreakpointsForDimension1=0:47  BreakpointsForDimension1FirstPoint=10  BreakpointsForDimension2FirstPoint=10  BreakpointsForDimension1Spacing=12  BreakpointsForDimension2Spacing=12  IndexSearchMethod=Evenly spaced points  Table=qam16  TableDataTypeStr=fixdt(0,4,0)  InterpMethod=Flat  DiagnosticForOutOfRangeInput=Error  InternalRulePriority=Speed  OutDataTypeStr=fixdt(0,4,0)  RndMeth=Simplest  InputSameDT=on
  HDL Counter : hdlsllib/Sources/HDL Counter  CountType=Count limited  CountInit=0  CountStep=1  CountMax=47  CountFromType=Initial value  CountFrom=0  CountResetPort=off  CountLoadPort=off  CountEnbPort=on  CountDirPort=off  CountDataType=Unsigned  CountWordLen=6  CountFracLen=0  CountSampTime=1
  bits : Outport  VectorParamsAs1DForOutWhenUnconnected=off
  validOut : Outport  Port=2  VectorParamsAs1DForOutWhenUnconnected=off
  wires:
  HDL Counter/1 -> 1-D Lookup Table/1
  ready/1 -> validOut/1, HDL Counter/1
  1-D Lookup Table/1 -> bits/1

== system OFDM_Tx_Rx_InterpDec/OFDMTx/DataGenerator/SymbolsGen/QPSKMap ==
  ints : Inport
  validIn : Inport  Port=2
  Constant : Constant  Value=1/sqrt(2) + 1/sqrt(2)*1i  VectorParams1D=off  OutDataTypeStr=fixdt(1,16,14)  SampleTime=1/fs
  Constant1 : Constant  Value=1/sqrt(2) - 1/sqrt(2)*1i  VectorParams1D=off  OutDataTypeStr=fixdt(1,16,14)  SampleTime=1/fs
  Constant2 : Constant  Value=-1/sqrt(2) + 1/sqrt(2)*1i  VectorParams1D=off  OutDataTypeStr=fixdt(1,16,14)  SampleTime=1/fs
  Constant3 : Constant  Value=-1/sqrt(2) - 1/sqrt(2)*1i  VectorParams1D=off  OutDataTypeStr=fixdt(1,16,14)  SampleTime=1/fs
  Constant4 : Constant  Value=complex(0)  VectorParams1D=off  OutDataTypeStr=fixdt(1,16,14)  SampleTime=1/fs
  Multiport Switch : MultiPortSwitch  DataPortOrder=Zero-based contiguous  Inputs=4  zeroidx=on
  Switch : Switch  Criteria=u2 ~= 0
  QPSKOut : Outport  VectorParamsAs1DForOutWhenUnconnected=off
  wires:
  Constant3/1 -> Multiport Switch/5
  Constant2/1 -> Multiport Switch/4
  ints/1 -> Multiport Switch/1
  Constant/1 -> Multiport Switch/2
  Constant1/1 -> Multiport Switch/3
  validIn/1 -> Switch/2
  Multiport Switch/1 -> Switch/1
  Constant4/1 -> Switch/3
  Switch/1 -> QPSKOut/1

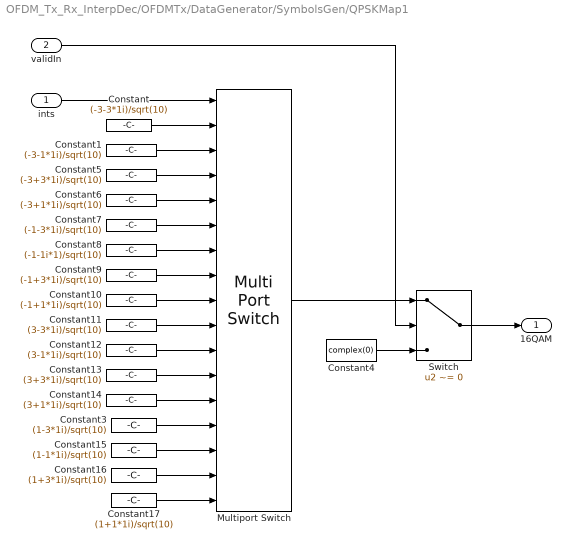
== system OFDM_Tx_Rx_InterpDec/OFDMTx/DataGenerator/SymbolsGen/QPSKMap1 ==
  ints : Inport
  validIn : Inport  Port=2
  Constant : Constant  Value=(-3-3*1i)/sqrt(10)  VectorParams1D=off  OutDataTypeStr=fixdt(1,16,14)  SampleTime=1/fs
  Constant1 : Constant  Value=(-3-1*1i)/sqrt(10)  VectorParams1D=off  OutDataTypeStr=fixdt(1,16,14)  SampleTime=1/fs
  Constant10 : Constant  Value=(-1+1*1i)/sqrt(10)  VectorParams1D=off  OutDataTypeStr=fixdt(1,16,14)  SampleTime=1/fs
  Constant11 : Constant  Value=(3-3*1i)/sqrt(10)  VectorParams1D=off  OutDataTypeStr=fixdt(1,16,14)  SampleTime=1/fs
  Constant12 : Constant  Value=(3-1*1i)/sqrt(10)  VectorParams1D=off  OutDataTypeStr=fixdt(1,16,14)  SampleTime=1/fs
  Constant13 : Constant  Value=(3+3*1i)/sqrt(10)  VectorParams1D=off  OutDataTypeStr=fixdt(1,16,14)  SampleTime=1/fs
  Constant14 : Constant  Value=(3+1*1i)/sqrt(10)  VectorParams1D=off  OutDataTypeStr=fixdt(1,16,14)  SampleTime=1/fs
  Constant15 : Constant  Value=(1-1*1i)/sqrt(10)  VectorParams1D=off  OutDataTypeStr=fixdt(1,16,14)  SampleTime=1/fs
  Constant16 : Constant  Value=(1+3*1i)/sqrt(10)  VectorParams1D=off  OutDataTypeStr=fixdt(1,16,14)  SampleTime=1/fs
  Constant17 : Constant  Value=(1+1*1i)/sqrt(10)  VectorParams1D=off  OutDataTypeStr=fixdt(1,16,14)  SampleTime=1/fs
  Constant3 : Constant  Value=(1-3*1i)/sqrt(10)  VectorParams1D=off  OutDataTypeStr=fixdt(1,16,14)  SampleTime=1/fs
  Constant4 : Constant  Value=complex(0)  VectorParams1D=off  OutDataTypeStr=fixdt(1,16,14)  SampleTime=1/fs
  Constant5 : Constant  Value=(-3+3*1i)/sqrt(10)  VectorParams1D=off  OutDataTypeStr=fixdt(1,16,14)  SampleTime=1/fs
  Constant6 : Constant  Value=(-3+1*1i)/sqrt(10)  VectorParams1D=off  OutDataTypeStr=fixdt(1,16,14)  SampleTime=1/fs
  Constant7 : Constant  Value=(-1-3*1i)/sqrt(10)  VectorParams1D=off  OutDataTypeStr=fixdt(1,16,14)  SampleTime=1/fs
  Constant8 : Constant  Value=(-1-1i*1)/sqrt(10)  VectorParams1D=off  OutDataTypeStr=fixdt(1,16,14)  SampleTime=1/fs
  Constant9 : Constant  Value=(-1+3*1i)/sqrt(10)  VectorParams1D=off  OutDataTypeStr=fixdt(1,16,14)  SampleTime=1/fs
  Multiport Switch : MultiPortSwitch  DataPortOrder=Zero-based contiguous  Inputs=16  zeroidx=on
  Switch : Switch  Criteria=u2 ~= 0
  16QAM : Outport  VectorParamsAs1DForOutWhenUnconnected=off
  wires:
  Switch/1 -> 16QAM/1
  Constant4/1 -> Switch/3
  Multiport Switch/1 -> Switch/1
  validIn/1 -> Switch/2
  ints/1 -> Multiport Switch/1
  Constant/1 -> Multiport Switch/2
  Constant1/1 -> Multiport Switch/3
  Constant5/1 -> Multiport Switch/4
  Constant6/1 -> Multiport Switch/5
  Constant7/1 -> Multiport Switch/6
  Constant8/1 -> Multiport Switch/7
  Constant9/1 -> Multiport Switch/8
  Constant10/1 -> Multiport Switch/9
  Constant11/1 -> Multiport Switch/10
  Constant12/1 -> Multiport Switch/11
  Constant13/1 -> Multiport Switch/12
  Constant14/1 -> Multiport Switch/13
  Constant3/1 -> Multiport Switch/14
  Constant15/1 -> Multiport Switch/15
  Constant16/1 -> Multiport Switch/16
  Constant17/1 -> Multiport Switch/17

== system OFDM_Tx_Rx_InterpDec/OFDMTx/IFFT/IFFTValid/dataIFFTValid ==
  dataValidIn : Inport
  Compare To Constant : simulink/Logic and Bit Operations/Compare To Constant  relop=>=  const=17  OutDataTypeStr=boolean
  Logical Operator : Logic  Operator=NOT  IconShape=distinctive  AllPortsSameDT=off  OutDataTypeStr=boolean
  SAMPLE_COUNTER : hdlsllib/Sources/HDL Counter  CountType=Count limited  CountInit=1  CountStep=1  CountMax=80  CountFromType=Initial value  CountFrom=1  CountResetPort=on  CountLoadPort=off  CountEnbPort=on  CountDirPort=off  CountDataType=Unsigned  CountWordLen=7  CountFracLen=0  CountSampTime=1
  dataIFFTValidOut : Outport  VectorParamsAs1DForOutWhenUnconnected=off
  wires:
  dataValidIn/1 -> SAMPLE_COUNTER/2, Logical Operator/1
  Compare To Constant/1 -> dataIFFTValidOut/1
  Logical Operator/1 -> SAMPLE_COUNTER/1
  SAMPLE_COUNTER/1 -> Compare To Constant/1

== system OFDM_Tx_Rx_InterpDec/OFDMTx/IFFT/IFFTValid/preambIFFTValid ==
  preambValid : Inport
  AND{,1..3} (4 alike) : Logic  IconShape=distinctive  AllPortsSameDT=off  OutDataTypeStr=boolean
  Compare To Constant1 : simulink/Logic and Bit Operations/Compare To Constant  relop=>=  const=96  OutDataTypeStr=boolean
  Compare To Constant2 : simulink/Logic and Bit Operations/Compare To Constant  relop=<=  const=159  OutDataTypeStr=boolean
  Compare To Constant3 : simulink/Logic and Bit Operations/Compare To Constant  relop=>=  const=256  OutDataTypeStr=boolean
  Compare To Constant4 : simulink/Logic and Bit Operations/Compare To Constant  relop=<=  const=319  OutDataTypeStr=boolean
  HDL Counter1 : hdlsllib/Sources/HDL Counter  CountType=Count limited  CountInit=0  CountStep=1  CountMax=319  CountFromType=Initial value  CountFrom=0  CountResetPort=on  CountLoadPort=off  CountEnbPort=on  CountDirPort=off  CountDataType=Unsigned  CountWordLen=9  CountFracLen=0  CountSampTime=1
  NOT : Logic  Operator=NOT  IconShape=distinctive  AllPortsSameDT=off  OutDataTypeStr=boolean
  OR : Logic  Operator=OR  IconShape=distinctive  AllPortsSameDT=off  OutDataTypeStr=boolean
  preambIFFTValidOut : Outport  VectorParamsAs1DForOutWhenUnconnected=off
  wires:
  AND/1 -> AND1/1
  AND2/1 -> AND3/1
  HDL Counter1/1 -> Compare To Constant4/1, Compare To Constant3/1, Compare To Constant2/1, Compare To Constant1/1
  OR/1 -> preambIFFTValidOut/1
  preambValid/1 -> HDL Counter1/2, AND3/2, AND1/2, NOT/1
  Compare To Constant1/1 -> AND/1
  Compare To Constant4/1 -> AND2/2
  AND1/1 -> OR/1
  AND3/1 -> OR/2
  Compare To Constant2/1 -> AND/2
  NOT/1 -> HDL Counter1/1
  Compare To Constant3/1 -> AND2/1

== system OFDM_Tx_Rx_InterpDec/OFDMTx/SCMapper/DataMapper/READ_CTRL2 ==
  In1 : Inport
  In2 : Inport  Port=2
  Constant : Constant  Value=0  OutDataTypeStr=fixdt(0,8,0)  SampleTime=1/fs
  Switch : Switch  Criteria=u2 ~= 0
  Out1 : Outport  VectorParamsAs1DForOutWhenUnconnected=off
  wires:
  Switch/1 -> Out1/1
  In1/1 -> Switch/1
  In2/1 -> Switch/2
  Constant/1 -> Switch/3

== system OFDM_Tx_Rx_InterpDec/OFDMTx/SCMapper/PremableMapper/READ_CTRL ==
  In1 : Inport
  In2 : Inport  Port=2
  Constant : Constant  Value=0  OutDataTypeStr=fixdt(0,8,0)  SampleTime=1/fs
  Switch : Switch  Criteria=u2 ~= 0
  Out1 : Outport  VectorParamsAs1DForOutWhenUnconnected=off
  wires:
  Switch/1 -> Out1/1
  In1/1 -> Switch/1
  In2/1 -> Switch/2
  Constant/1 -> Switch/3

== system OFDM_Tx_Rx_InterpDec/OFDMRx/PhaseTracking/PilotCtrlGen/pilotGen/ToComplex1 ==
  In1 : Inport
  Constant1 : Constant  Value=0  OutDataTypeStr=fixdt(1,2,0)  SampleTime=1/fs
  Real-Imag to Complex : RealImagToComplex
  Out1 : Outport  VectorParamsAs1DForOutWhenUnconnected=off
  wires:
  Real-Imag to Complex/1 -> Out1/1
  In1/1 -> Real-Imag to Complex/1
  Constant1/1 -> Real-Imag to Complex/2

== system OFDM_Tx_Rx_InterpDec/OFDMRx/Synchronisation/CoarseTimingSynch/CoarseTimeStrobeGen/LocalSearchCounter ==
  note: Counter starts at 0
  note: Sample counter which is for local serach of X samples
      | after frame starting point. The counter resets
      | after X samples and is only initiated when the frame
      | detection pulse goes HIGH.
  packDetIn : Inport
  Compare To Constant : simulink/Logic and Bit Operations/Compare To Constant  relop===  const=19  OutDataTypeStr=boolean
  Constant : Constant  OutDataTypeStr=boolean  SampleTime=1/fs
  HDL Counter : hdlsllib/Sources/HDL Counter  CountType=Count limited  CountInit=0  CountStep=1  CountMax=19  CountFromType=Initial value  CountFrom=0  CountResetPort=on  CountLoadPort=off  CountEnbPort=on  CountDirPort=off  CountDataType=Unsigned  CountWordLen=8  CountFracLen=0  CountSampTime=1
  NOT : Logic  Operator=NOT  IconShape=distinctive  AllPortsSameDT=off  OutDataTypeStr=boolean
  RsingEdge : Subsystem
  Unit Delay Enabled Resettable Synchronous : hdlsllib/Discrete/Unit Delay Enabled Resettable Synchronous  InitialCondition=0.0  SampleTime=-1
      settings: SourceProductBaseCode=SL
  coutEnb : Outport  VectorParamsAs1DForOutWhenUnconnected=off
  countOut : Outport  Port=2  VectorParamsAs1DForOutWhenUnconnected=off
  wires:
  Unit Delay Enabled Resettable Synchronous/1 -> NOT/1, HDL Counter/2, coutEnb/1
  Compare To Constant/1 -> Unit Delay Enabled Resettable Synchronous/3
  Constant/1 -> Unit Delay Enabled Resettable Synchronous/1
  HDL Counter/1 -> Compare To Constant/1, countOut/1
  RsingEdge/1(Out1) -> Unit Delay Enabled Resettable Synchronous/2
  packDetIn/1 -> RsingEdge/1(In1)
  NOT/1 -> HDL Counter/1

== system OFDM_Tx_Rx_InterpDec/OFDMRx/Synchronisation/CoarseTimingSynch/CoarseTimeStrobeGen/MaxPeakDet ==
  note: After the maximum value in the window of X samples has
      | been found, the index of the maximum is compared to the
      | output of a counter. The point where the counter equals the
      | index of the maximum is the coarse timing point plus a delay
      | of X samples. This delay must be compensated on all parallel
      | signal paths.
  note: This register records the counter value for the sample
      | with the maximum value i.e. its index
  note: Register updates every time a new maximum value is
      | found inside the window of X samples after the point where
      | a valid frame is found.
  DataIn : Inport
  CntEnbIn : Inport  Port=2
  CountIn : Inport  Port=3
  Delay2 : Delay  DelayLength=20
  Delay3 : Delay  DelayLength=1
  Delay5 : Delay  DelayLength=20
  Delay6 : Delay  DelayLength=1
  Logical Operator : Logic  IconShape=distinctive  AllPortsSameDT=off  OutDataTypeStr=boolean
  Logical Operator1 : Logic  IconShape=distinctive  AllPortsSameDT=off  OutDataTypeStr=boolean
  Relational Operator : RelationalOperator  Operator=>  OutDataTypeStr=boolean  RndMeth=Nearest
  Relational Operator1 : RelationalOperator  Operator===  OutDataTypeStr=boolean  RndMeth=Nearest
  Unit Delay Enabled Synchronous : hdlsllib/Discrete/Unit Delay Enabled Synchronous  InitialCondition=0.0  SampleTime=-1
      settings: SourceProductBaseCode=SL
  Unit Delay Enabled Synchronous1 : hdlsllib/Discrete/Unit Delay Enabled Synchronous  InitialCondition=0.0  SampleTime=-1
      settings: SourceProductBaseCode=SL
  CoarseStrbOut : Outport  VectorParamsAs1DForOutWhenUnconnected=off
  wires:
  Logical Operator1/1 -> CoarseStrbOut/1
  CountIn/1 -> Delay5/1, Unit Delay Enabled Synchronous1/1
  CntEnbIn/1 -> Delay2/1, Logical Operator/2
  Delay5/1 -> Delay6/1
  Unit Delay Enabled Synchronous/1 -> Relational Operator/2
  Unit Delay Enabled Synchronous1/1 -> Relational Operator1/1
  Relational Operator1/1 -> Logical Operator1/2
  Delay3/1 -> Logical Operator1/1
  Delay2/1 -> Delay3/1
  Relational Operator/1 -> Logical Operator/1
  DataIn/1 -> Unit Delay Enabled Synchronous/1, Relational Operator/1
  Logical Operator/1 -> Unit Delay Enabled Synchronous/2, Unit Delay Enabled Synchronous1/2
  Delay6/1 -> Relational Operator1/2

== system OFDM_Tx_Rx_InterpDec/OFDMRx/Synchronisation/ControlSigGen/PreambleValidGen/RisingEdge ==
  ValidIn : Inport
  Delay : Delay  DelayLength=1
  Relational Operator : RelationalOperator  Operator=>  OutDataTypeStr=boolean  RndMeth=Nearest
  Out1 : Outport
  wires:
  Relational Operator/1 -> Out1/1
  Delay/1 -> Relational Operator/2
  ValidIn/1 -> Delay/1, Relational Operator/1

== system OFDM_Tx_Rx_InterpDec/OFDMRx/Synchronisation/FineTimingSynch/MatchedFilter/Adder ==
  In1 : Inport
  In2 : Inport  Port=2
  Add : Sum  AccumDataTypeStr=fixdt(1,24,14)
  Delay3 : Delay  DelayLength=1
  Out1 : Outport  VectorParamsAs1DForOutWhenUnconnected=off
  wires:
  In2/1 -> Delay3/1
  In1/1 -> Add/1
  Add/1 -> Out1/1
  Delay3/1 -> Add/2

== system OFDM_Tx_Rx_InterpDec/OFDMRx/Synchronisation/FineTimingSynch/MatchedFilter/Adder1 ==
  In1 : Inport
  In2 : Inport  Port=2
  Add : Sum  AccumDataTypeStr=fixdt(1,24,14)
  Delay3 : Delay  DelayLength=1
  Out1 : Outport  VectorParamsAs1DForOutWhenUnconnected=off
  wires:
  Delay3/1 -> Add/2
  Add/1 -> Out1/1
  In1/1 -> Add/1
  In2/1 -> Delay3/1

== system OFDM_Tx_Rx_InterpDec/OFDMRx/Synchronisation/FineTimingSynch/MatchedFilter/Adder10 ==
  In1 : Inport
  In2 : Inport  Port=2
  Add : Sum  AccumDataTypeStr=fixdt(1,24,14)
  Delay3 : Delay  DelayLength=1
  Out1 : Outport  VectorParamsAs1DForOutWhenUnconnected=off
  wires:
  In2/1 -> Delay3/1
  In1/1 -> Add/1
  Add/1 -> Out1/1
  Delay3/1 -> Add/2

== system OFDM_Tx_Rx_InterpDec/OFDMRx/Synchronisation/FineTimingSynch/MatchedFilter/Adder11 ==
  In1 : Inport
  In2 : Inport  Port=2
  Add : Sum  AccumDataTypeStr=fixdt(1,24,14)
  Delay3 : Delay  DelayLength=1
  Out1 : Outport  VectorParamsAs1DForOutWhenUnconnected=off
  wires:
  Delay3/1 -> Add/2
  Add/1 -> Out1/1
  In1/1 -> Add/1
  In2/1 -> Delay3/1

== system OFDM_Tx_Rx_InterpDec/OFDMRx/Synchronisation/FineTimingSynch/MatchedFilter/Adder12 ==
  In1 : Inport
  In2 : Inport  Port=2
  Add : Sum  AccumDataTypeStr=fixdt(1,24,14)
  Delay3 : Delay  DelayLength=1
  Out1 : Outport  VectorParamsAs1DForOutWhenUnconnected=off
  wires:
  In2/1 -> Delay3/1
  In1/1 -> Add/1
  Add/1 -> Out1/1
  Delay3/1 -> Add/2

== system OFDM_Tx_Rx_InterpDec/OFDMRx/Synchronisation/FineTimingSynch/MatchedFilter/Adder13 ==
  In1 : Inport
  In2 : Inport  Port=2
  Add : Sum  AccumDataTypeStr=fixdt(1,24,14)
  Delay3 : Delay  DelayLength=1
  Out1 : Outport  VectorParamsAs1DForOutWhenUnconnected=off
  wires:
  Delay3/1 -> Add/2
  Add/1 -> Out1/1
  In1/1 -> Add/1
  In2/1 -> Delay3/1

== system OFDM_Tx_Rx_InterpDec/OFDMRx/Synchronisation/FineTimingSynch/MatchedFilter/Adder14 ==
  In1 : Inport
  In2 : Inport  Port=2
  Add : Sum  AccumDataTypeStr=fixdt(1,24,14)
  Delay3 : Delay  DelayLength=1
  Out1 : Outport  VectorParamsAs1DForOutWhenUnconnected=off
  wires:
  In2/1 -> Delay3/1
  In1/1 -> Add/1
  Add/1 -> Out1/1
  Delay3/1 -> Add/2

== system OFDM_Tx_Rx_InterpDec/OFDMRx/Synchronisation/FineTimingSynch/MatchedFilter/Adder15 ==
  In1 : Inport
  In2 : Inport  Port=2
  Add : Sum  AccumDataTypeStr=fixdt(1,24,14)
  Delay3 : Delay  DelayLength=1
  Out1 : Outport  VectorParamsAs1DForOutWhenUnconnected=off
  wires:
  Delay3/1 -> Add/2
  Add/1 -> Out1/1
  In1/1 -> Add/1
  In2/1 -> Delay3/1

== system OFDM_Tx_Rx_InterpDec/OFDMRx/Synchronisation/FineTimingSynch/MatchedFilter/Adder16 ==
  In1 : Inport
  In2 : Inport  Port=2
  Add : Sum  AccumDataTypeStr=fixdt(1,24,14)
  Delay3 : Delay  DelayLength=1
  Out1 : Outport  VectorParamsAs1DForOutWhenUnconnected=off
  wires:
  In2/1 -> Delay3/1
  In1/1 -> Add/1
  Add/1 -> Out1/1
  Delay3/1 -> Add/2

== system OFDM_Tx_Rx_InterpDec/OFDMRx/Synchronisation/FineTimingSynch/MatchedFilter/Adder17 ==
  In1 : Inport
  In2 : Inport  Port=2
  Add : Sum  AccumDataTypeStr=fixdt(1,24,14)
  Delay3 : Delay  DelayLength=1
  Out1 : Outport  VectorParamsAs1DForOutWhenUnconnected=off
  wires:
  Delay3/1 -> Add/2
  Add/1 -> Out1/1
  In1/1 -> Add/1
  In2/1 -> Delay3/1

== system OFDM_Tx_Rx_InterpDec/OFDMRx/Synchronisation/FineTimingSynch/MatchedFilter/Adder18 ==
  In1 : Inport
  In2 : Inport  Port=2
  Add : Sum  AccumDataTypeStr=fixdt(1,24,14)
  Delay3 : Delay  DelayLength=1
  Out1 : Outport  VectorParamsAs1DForOutWhenUnconnected=off
  wires:
  In2/1 -> Delay3/1
  In1/1 -> Add/1
  Add/1 -> Out1/1
  Delay3/1 -> Add/2

== system OFDM_Tx_Rx_InterpDec/OFDMRx/Synchronisation/FineTimingSynch/MatchedFilter/Adder19 ==
  In1 : Inport
  In2 : Inport  Port=2
  Add : Sum  AccumDataTypeStr=fixdt(1,24,14)
  Delay3 : Delay  DelayLength=1
  Out1 : Outport  VectorParamsAs1DForOutWhenUnconnected=off
  wires:
  In2/1 -> Delay3/1
  In1/1 -> Add/1
  Add/1 -> Out1/1
  Delay3/1 -> Add/2

== system OFDM_Tx_Rx_InterpDec/OFDMRx/Synchronisation/FineTimingSynch/MatchedFilter/Adder2 ==
  In1 : Inport
  In2 : Inport  Port=2
  Add : Sum  AccumDataTypeStr=fixdt(1,24,14)
  Delay3 : Delay  DelayLength=1
  Out1 : Outport  VectorParamsAs1DForOutWhenUnconnected=off
  wires:
  In2/1 -> Delay3/1
  In1/1 -> Add/1
  Add/1 -> Out1/1
  Delay3/1 -> Add/2

== system OFDM_Tx_Rx_InterpDec/OFDMRx/Synchronisation/FineTimingSynch/MatchedFilter/Adder20 ==
  In1 : Inport
  In2 : Inport  Port=2
  Add : Sum  AccumDataTypeStr=fixdt(1,24,14)
  Delay3 : Delay  DelayLength=1
  Out1 : Outport  VectorParamsAs1DForOutWhenUnconnected=off
  wires:
  In2/1 -> Delay3/1
  In1/1 -> Add/1
  Add/1 -> Out1/1
  Delay3/1 -> Add/2

== system OFDM_Tx_Rx_InterpDec/OFDMRx/Synchronisation/FineTimingSynch/MatchedFilter/Adder21 ==
  In1 : Inport
  In2 : Inport  Port=2
  Add : Sum  AccumDataTypeStr=fixdt(1,24,14)
  Delay3 : Delay  DelayLength=1
  Out1 : Outport  VectorParamsAs1DForOutWhenUnconnected=off
  wires:
  In2/1 -> Delay3/1
  In1/1 -> Add/1
  Add/1 -> Out1/1
  Delay3/1 -> Add/2
